simulink model "IntegratedBehaviorModule"  (R2024b)
settings: Solver=VariableStepAuto  StartTime=0.0  StopTime=inf  RelTol=1e-3
StartFcn:
  | clf
model workspace (MAT data in the model file):
  SL_ROS_VariableLengthArrays_MaxSizes : object (value not decoded)
  Sig : Simulink.Signal (value not decoded)
undefined symbols (not defined in the file or in its folder): dem, fixedTEBParams, goalPose, initialTranslationTruck, mapSize, maxRefPathLen, nlobjTracking, pathBus_struct, TaskControllerModeType, tuneableTEBParamsCpp, tuneableTerrainAwareParams, worldGridLoc, worldMat, worldRes
libraries: simulink x10, roshelperlib x5, robotmobilelib x1, robotsim3dlib x1, sim3dlib x1
(part 2 of 2)

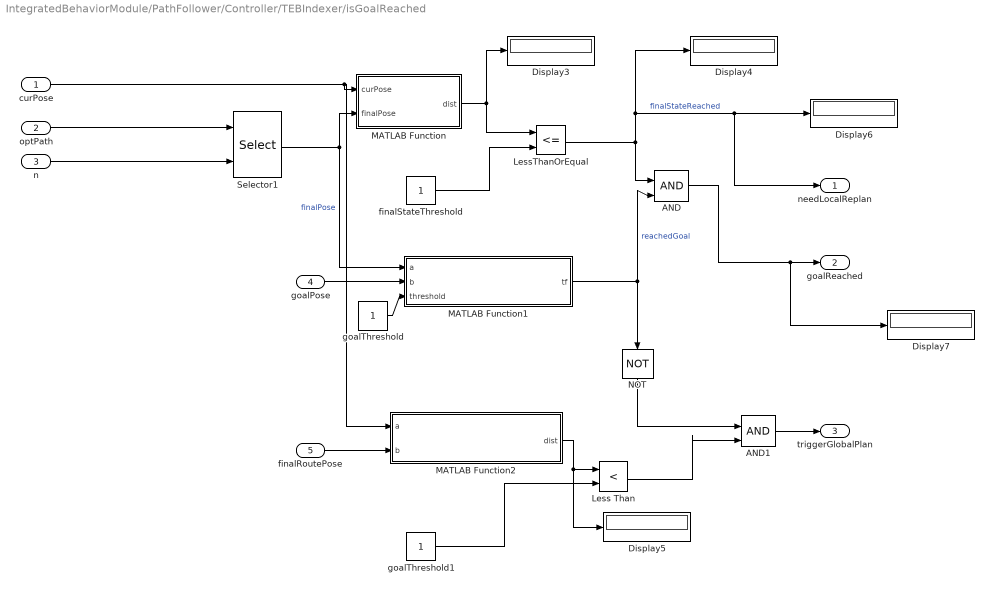
== system IntegratedBehaviorModule/PathFollower/Controller/TEBIndexer/isGoalReached ==
  curPose : Inport
  optPath : Inport  Port=2
  n : Inport  Port=3
  goalPose : Inport  Port=4
  finalRoutePose : Inport  Port=5
  AND : Logic  IconShape=distinctive  AllPortsSameDT=off  OutDataTypeStr=boolean
  AND1 : Logic  IconShape=distinctive  AllPortsSameDT=off  OutDataTypeStr=boolean
  Display{3..7} (5 alike) : Display
  Less Than : RelationalOperator  Operator=<  OutDataTypeStr=boolean  RndMeth=Simplest  InputSameDT=off
  LessThanOrEqual : RelationalOperator  Operator=<=  OutDataTypeStr=boolean  RndMeth=Simplest  InputSameDT=off
  MATLAB Function : MATLAB Function  TreatAsAtomicUnit=on
  MATLAB Function1 : MATLAB Function  TreatAsAtomicUnit=on
  MATLAB Function2 : MATLAB Function  TreatAsAtomicUnit=on
  NOT : Logic  Operator=NOT  IconShape=distinctive  AllPortsSameDT=off  OutDataTypeStr=boolean
  Selector1 : Selector  NumberOfDimensions=2  InputPortWidth=1  IndexOptions=Index vector (port),Select all  Indices=[1 3],1  OutputSizes=1,1
  finalStateThreshold : Constant
  goalThreshold : Constant
  goalThreshold1 : Constant
  needLocalReplan : Outport
  goalReached : Outport  Port=2
  triggerGlobalPlan : Outport  Port=3
  wires:
  curPose/1 -> MATLAB Function2/1(a), MATLAB Function/1(curPose)
  optPath/1 -> Selector1/1
  Selector1/1 -> MATLAB Function1/1(a), MATLAB Function/2(finalPose)  "finalPose"
  finalStateThreshold/1 -> LessThanOrEqual/2
  LessThanOrEqual/1 -> Display4/1, needLocalReplan/1, Display6/1, AND/1  "finalStateReached"
  goalPose/1 -> MATLAB Function1/2(b)
  MATLAB Function1/1(tf) -> AND/2, NOT/1  "reachedGoal"
  AND/1 -> Display7/1, goalReached/1
  MATLAB Function/1(dist) -> Display3/1, LessThanOrEqual/1
  n/1 -> Selector1/2
  goalThreshold/1 -> MATLAB Function1/3(threshold)
  finalRoutePose/1 -> MATLAB Function2/2(b)
  NOT/1 -> AND1/1
  AND1/1 -> triggerGlobalPlan/1
  goalThreshold1/1 -> Less Than/2
  Less Than/1 -> AND1/2
  MATLAB Function2/1(dist) -> Display5/1, Less Than/1

== stateflow chart IntegratedBehaviorModule/TaskController ==
  state WaitingForTask
    entry:
    waitForTask = true;
    exit:
    waitForTask = false;
  state RoutePlanner
    entry:
    curGoal = newGoal;
    send(planRoute);
    planning = 0;
  state LocalPlanner
    entry:
    send(planLocal);
    planning = 0;
  state FollowingPath
    entry:
    followPath = true;
    exit:
    followPath = false;
  state GlobalPlanner
    entry:
    send(planGlobal);
    planning = 0;
  (default) -> WaitingForTask
  (junction 52) -> WaitingForTask
  FollowingPath -> (junction 52) [order 1] : [hasReachedGoal]
      | {waitForTask = true;}
  WaitingForTask -> RoutePlanner : [~isWaiting && ~any(isnan(newGoal))]
  RoutePlanner -> LocalPlanner : [~planning]
  LocalPlanner -> FollowingPath [order 1] : [~planning]
  FollowingPath -> LocalPlanner [order 3] : [needLocalReplan]
  LocalPlanner -> GlobalPlanner [order 2] : [needGlobalReplan]
  GlobalPlanner -> LocalPlanner : [~planning]
  FollowingPath -> (junction 54) [order 2] : [needGlobalReplan]
  (junction 54) -> GlobalPlanner
  data: isWaiting input; newGoal input; needGlobalReplan input; needLocalReplan input; hasReachedGoal input; waitForTask output boolean; followPath output boolean; curGoal output size=[1 3]; planning local; TaskControllerMode output Enum: TaskControllerModeType
  events: planLocal output FUNCTION_CALL_EVENT; planRoute output FUNCTION_CALL_EVENT; planGlobal output FUNCTION_CALL_EVENT

== matlab function IntegratedBehaviorModule/PathFollower/Controller/TEBIndexer/isGoalReached/MATLAB Function ==
  data: curPose input; dist output; finalPose input
function dist = fcn(curPose, finalPose)
    dist = norm([curPose(1:2)-finalPose(1:2) angdiff(curPose(3),finalPose(3))],2);
end

== matlab function IntegratedBehaviorModule/PathFollower/Controller/TEBMPCCascade/MATLAB Function ==
  data: prevPath input; curPath output; curPath input; pathChanged output; n input
function [curPath,pathChanged] = didPathChange(prevPath, curPath, n)
    pathChanged = double(~isequal(curPath(1:n,:),prevPath(1:n,:)));
end

== matlab function IntegratedBehaviorModule/Operational Status/Simulink Signals/Confirm New Goal/compareToPrevious ==
  data: curGoal input; isNewGoal output; newGoal input
function isNewGoal = newGoalProvided(curGoal,newGoal)
    isNewGoal = ~isequal(curGoal,newGoal) && ~isequal(newGoal,zeros(1,3));
end

== matlab function IntegratedBehaviorModule/PathFollower/Controller/TEBIndexer/isGoalReached/MATLAB Function1 ==
  data: a input; tf output; b input; threshold input
function tf = reachedGoalFcn(a,b,threshold)
    tf = norm(a-b,2) < threshold;
end

== matlab function IntegratedBehaviorModule/PathFollower/Controller/TEBIndexer/isGoalReached/MATLAB Function2 ==
  data: a input; dist output; b input
function dist = reachedRouteEndFcn(a,b)
    dist = norm([a(1:2)-b(1:2) angdiff(a(3),b(3))]);
end

== matlab function IntegratedBehaviorModule/PathFollower/Controller/TEBMPCCascade/MATLAB Function1 ==
  data: prevMPCCmd input; curVel input; velcmd output; wheelBase input
function velcmd = vel2mpc(prevMPCCmd,curVel,wheelBase)
velcmd = curVel;
if velcmd(1) == 0
    % Use previous steering angle when velocity is 0
    velcmd(2) = prevMPCCmd(2);
else
    % Otherwise compute it from turn-rate
    velcmd(2) = atan(curVel(2)*wheelBase/velcmd(1));
end

== matlab function IntegratedBehaviorModule/EnvironmentSensorProcessing/Platform Model/Unreal (3D)/MATLAB Function1 ==
  data: curVel input; velcmd output; wheelBase input; prevMPCCmd input
function velcmd = vel2mpc(curVel,wheelBase,prevMPCCmd)
velcmd = curVel;
if velcmd(1) == 0
    % Use previous steering angle when velocity is 0
    velcmd(2) = prevMPCCmd(2);
else
    % Otherwise compute it from turn-rate
    velcmd(2) = atan(curVel(2)*wheelBase/velcmd(1));
end

== stateflow chart IntegratedBehaviorModule/PathFollower/Controller/TEBMPCCascade/Chart ==
  (default) -> (junction 11) : {
      | needLocalReplan = 0;
      | needGlobalPlan = 0;
      | goalReached = 0;
      | goalThreshold = 1;
      | }
  (junction 11) -> (junction 13) [order 1] : [poseReached(curPose,goalPose,goalThreshold,0.5)]
      | {goalReached = 1;}
  (junction 11) -> (junction 15) [order 2]
  (junction 13) -> (junction 26)
  (junction 15) -> (junction 26) [order 1] : [poseReached(curPose,finalPathPose,goalThreshold,0)]
      | {needGlobalPlan = 1;}
  (junction 15) -> (junction 33) [order 2] : {velcmd = mpcVelCmd;}
  (junction 26) -> (junction 28)
  (junction 33) -> (junction 35) [order 1] : [poseReached(curPose,segmentEndPose,goalThreshold,0)]
  (junction 35) -> (junction 28) [order 1] : [nMPCRefRows - nearestIdx <= mpcNumTS]
      | {needLocalReplan = 1;}
  (junction 28) -> (junction 30) : {velcmd = [0 0];}
  (junction 33) -> (junction 30) [order 2]
  (junction 35) -> (junction 30) [order 2]
  data: pose function_input; targetPose function_input; threshold function_input; orientationWeight function_input; isReached function_output; nMPCRefRows input; nearestIdx input; mpcNumTS input; needLocalReplan output; needGlobalPlan output; curPose input; segmentEndPose input; finalPathPose input; goalPose input; goalReached output; velcmd output; goalThreshold local; mpcVelCmd input
  function isReached = poseReached(pose,targetPose,threshold,orientationWeight):
    | function isReached = poseReached(pose,targetPose,threshold,orientationWeight)
    |     arguments
    |         pose (1,3)
    |         targetPose (1,3)
    |         threshold (1,1) {mustBePositive} = 1;
    |         orientationWeight (1,1) {mustBeInRange(orientationWeight,0,1)} = 0;
    |     end
    |     dv = (pose-targetPose);
    |     dist = norm(dv.* [1 1 orientationWeight],2);
    |     isReached = dist <= threshold;
    | end
